simulink model "digifilter"  (R2021b)
settings: Solver=VariableStepAuto  StartTime=0.0  StopTime=500e-6  RelTol=1e-3
settings Model: Creator=Chris  LastModifiedBy=casey
settings SolverCC: AlgebraicLoopSolver=TrustRegion
settings DataIOCC: ReturnWorkspaceOutputs=off
settings DebuggingCC: SFMachineParentedDataDiag=warning  ArithmeticOperatorsInVariantConditions=warning
settings SFSimCC: SimUseLocalCustomCode=off  CustomCodeUndefinedFunction=UseInterfaceOnly
settings RTWCC: RTWUseLocalCustomCode=off  DLArmComputeVersion=20.02.1

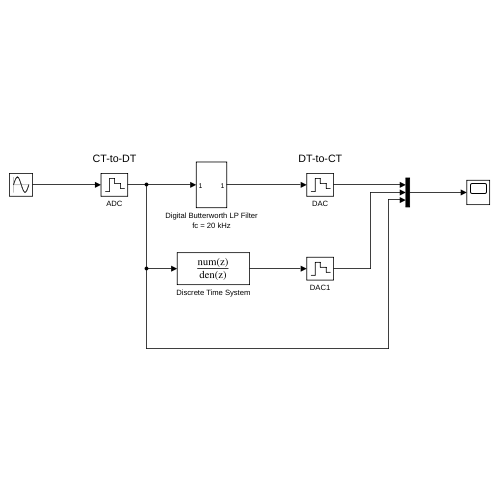
[thumbnail: Simulink's stored preview of the top-level diagram]
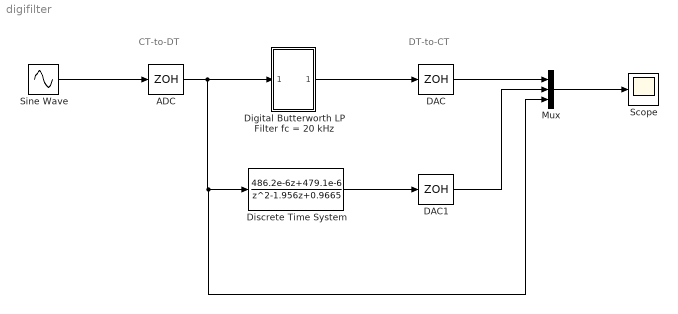
== system digifilter ==
  note: DT-to-CT
  note: CT-to-DT
  ADC : ZeroOrderHold  SampleTime=0.25e-6
  DAC : ZeroOrderHold  SampleTime=0.25e-6
  DAC1 : ZeroOrderHold  SampleTime=0.25e-6
  Digital Butterworth LP Filter fc = 20 kHz : Subsystem
  Discrete Time System : DiscreteTransferFcn  Numerator=[0 486.2e-6 479.1e-6]  Denominator=[1 -1.956 0.9665]
  Mux : Mux  Inputs=3
  Scope : Scope
  Sine Wave : Sin  Frequency=0.1*1.2566e+05  SampleTime=0
  wires:
  Sine Wave/1 -> ADC/1
  ADC/1 -> Mux/3, Discrete Time System/1, Digital Butterworth LP Filter fc = 20 kHz/1(In1)
  Digital Butterworth LP Filter fc = 20 kHz/1(Out1) -> DAC/1
  Discrete Time System/1 -> DAC1/1
  DAC/1 -> Mux/1
  Mux/1 -> Scope/1
  DAC1/1 -> Mux/2

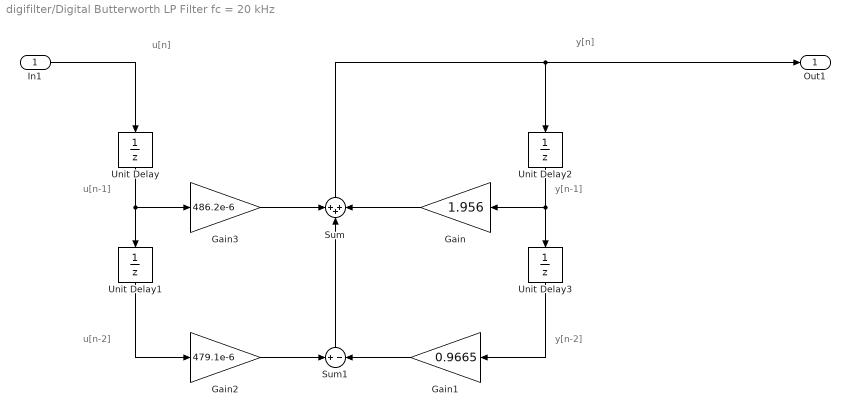
== system digifilter/Digital Butterworth LP Filter fc = 20 kHz ==
  note: y[n-2]
  note: y[n-1]
  note: y[n]
  note: u[n-2]
  note: u[n-1]
  note: u[n]
  In1 : Inport
  Gain : Gain  Gain=1.956
  Gain1 : Gain  Gain=0.9665
  Gain2 : Gain  Gain=479.1e-6
  Gain3 : Gain  Gain=486.2e-6
  Sum : Sum  Inputs=+++
  Sum1 : Sum  Inputs=+|-
  Unit Delay{,1..3} (4 alike) : UnitDelay  SampleTime=-1  HasFrameUpgradeWarning=on
  Out1 : Outport  VectorParamsAs1DForOutWhenUnconnected=off
  wires:
  Sum1/1 -> Sum/2
  Gain3/1 -> Sum/1
  Unit Delay/1 -> Gain3/1, Unit Delay1/1
  Gain/1 -> Sum/3
  Unit Delay2/1 -> Unit Delay3/1, Gain/1
  Unit Delay3/1 -> Gain1/1
  Unit Delay1/1 -> Gain2/1
  Gain2/1 -> Sum1/1
  Sum/1 -> Out1/1, Unit Delay2/1
  Gain1/1 -> Sum1/2
  In1/1 -> Unit Delay/1
